simulink model "buckwithmppt"  (R2020b)
settings: Solver=ode23t  StartTime=0.0  StopTime=0.5  RelTol=1e-3
libraries: powerlib x9, re_lib x1, eePwmGenerator x1
settings Model: Creator=shashank Pathak  LastModifiedBy=shashank Pathak

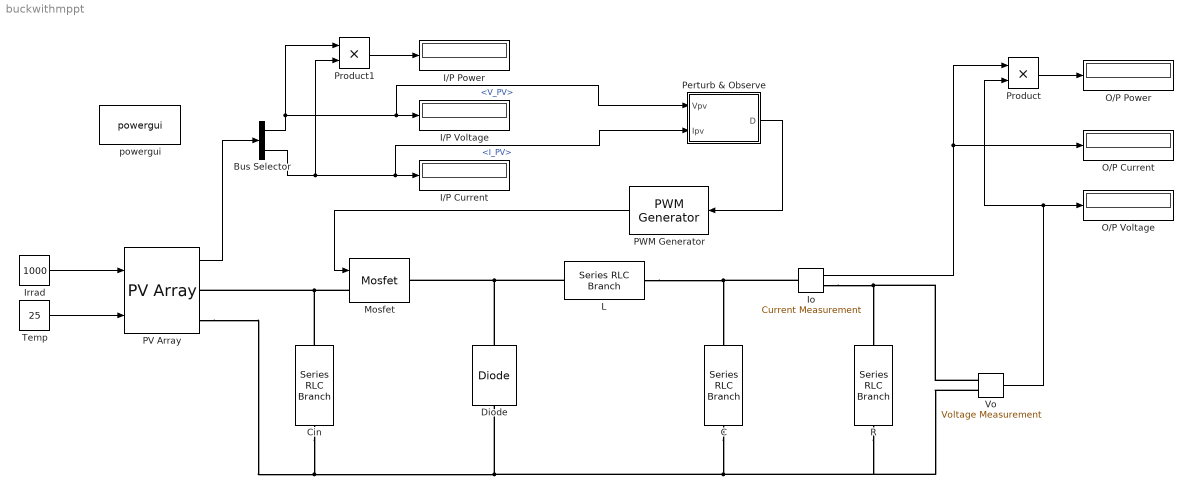
== system buckwithmppt ==
  Bus Selector : BusSelector  OutputSignals=V_PV,I_PV
  C : powerlib/Elements/Series RLC Branch  LConnTagsString=__new0  RConnTagsString=__new0  BranchType=C  Resistance=1  Inductance=1e-3  SetiL0=off  InitialCurrent=0  Capacitance=2.502e-6  Setx0=off  InitialVoltage=0  Measurements=None
  Cin : powerlib/Elements/Series RLC Branch  LConnTagsString=__new0  RConnTagsString=__new0  BranchType=RC  Resistance=0.0001  Inductance=1e-3  SetiL0=off  InitialCurrent=0  Capacitance=1000e-6  Setx0=off  InitialVoltage=0  Measurements=None
  Diode : powerlib/Power Electronics/Diode  Ron=0.001  Lon=0  Vf=0.8  IC=0  UseSnubber=0  Rs=500  Cs=250e-9  Measurements=off
  I/P Current : Display
  I/P Power : Display
  I/P Voltage : Display
  Io : powerlib/Measurements/Current Measurement  PhasorSimulation=off  OutputType=Complex  PSBequivalent=0
  Irrad : Constant  Value=1000
  L : powerlib/Elements/Series RLC Branch  LConnTagsString=__new0  RConnTagsString=__new0  BranchType=L  Resistance=1  Inductance=9.92e-5  SetiL0=off  InitialCurrent=0  Capacitance=1e-6  Setx0=off  InitialVoltage=0  Measurements=None
  Mosfet : powerlib/Power Electronics/Mosfet  Ron=0.1  Lon=0  Rd=0.01  Vfd=0  IC=0  Rs=1e5  Cs=inf  Measurements=off
  O/P Current : Display
  O/P Power : Display
  O/P Voltage : Display
  PV Array : re_lib/Solar/PV Array  Npar=1  Nser=1  PlotType=array @ 25 deg.C & specified irradiances  S_vec=[ 1000 500 100 ]  Temp_C_vec="[ 45 25  ]"  ModuleName=User-defined  PlotWhenSelected=off  Pm=213.15  Ncell=60  Voc=36.3  Isc=7.84  Vm=29  Im=7.35  beta_Voc_pc=-0.36099  alpha_Isc_pc=0.102  beta_Voc=-0.13104  alpha_Isc=0.0079968  IL=7.8654  I0=2.9273e-10  nI=0.98119  Rsh=313.0553  Rs=0.39381  RobustModel=off  RobustCellTemperature=313.3991  BAL=on  Tc=1e-6  Tfilter=5e-5
  PWM Generator : eePwmGenerator/PWM Generator  CarrCount=Up  Tper=1/5000  Ts=10e-6
  Perturb & Observe : MATLAB Function  TreatAsAtomicUnit=on
  Product : Product
  Product1 : Product
  R : powerlib/Elements/Series RLC Branch  LConnTagsString=__new0  RConnTagsString=__new0  BranchType=R  Resistance=1  Inductance=1e-3  SetiL0=off  InitialCurrent=0  Capacitance=1e-6  Setx0=off  InitialVoltage=0  Measurements=None
  Temp : Constant  Value=25
  Vo : powerlib/Measurements/Voltage Measurement  PhasorSimulation=off  OutputType=Complex  PSBequivalent=0
  powergui : powerlib/powergui  Priority=1  SimulationMode=Discrete  SampleTime=1e-6  frequency=60  Iterations=50  frequencyindice=0  Pbase=100e6  ErrMax=1e-4  UnitsV=kV  UnitsW=MW  buscounter=0  FunctionMessages=off  echomessages=off  EnableUseOfTLC=off  CurrentSourceSwitches=off  DisableSnubberDevices=off  DisableRonSwitches=off  DisableVfSwitches=off  DisplayEquations=off  AutomaticDiscreteSolvers=off  SolverType=Tustin/Backward Euler (TBE)  Interpol=off  ExternalGateDelay=off  methode=off  Ts=100  x0status=blocks  SPID=on  SwTol=0  HookPort=off  NonlinearTolerance=1e-4  nMaxIteration=100  ContinueOnMaxIteration=off  RestoreLinks=warning  ResistiveCurrentMeasurement=off  Frange=[0:2:500]  Ylog=off  Xlog=on  ShowGrid=off  save=off  variable=ZData  structure=0  ZoomFFT=off  StartTime=0.0  cycles=1  DisplayStyle=1  fundamental=60  FreqAxis=off  MaxFrequency=1000  frequencyindicesteady=1  RmsSteady=1  display=off
  wires:
  Irrad/1 -> PV Array/1
  Temp/1 -> PV Array/2
  PV Array/1 -> Bus Selector/1
  Bus Selector/1 -> Product1/1, I/P Voltage/1, Perturb & Observe/1(Vpv)  "<V_PV>"
  Bus Selector/2 -> Product1/2, Perturb & Observe/2(Ipv), I/P Current/1  "<I_PV>"
  Io/1 -> Product/1, O/P Current/1
  Vo/1 -> Product/2, O/P Voltage/1
  Product/1 -> O/P Power/1
  Product1/1 -> I/P Power/1
  PWM Generator/1 -> Mosfet/1
  Perturb & Observe/1(D) -> PWM Generator/1
  connections:
  Mosfet/LConn1 -- Cin/LConn1 -- PV Array/RConn1
  L/LConn1 -- Mosfet/RConn1 -- Diode/RConn1
  L/RConn1 -- Io/LConn1 -- C/LConn1
  PV Array/RConn2 -- Cin/RConn1 -- R/RConn1 -- Vo/LConn2 -- C/RConn1 -- Diode/LConn1
  Io/RConn1 -- Vo/LConn1 -- R/LConn1

== matlab function buckwithmppt/Perturb & Observe ==
  data: Vpv input; D output; Ipv input
function D = PO(Vpv, Ipv)

persistent Dprev Vprev Pprev

if isempty(Dprev)
    Dprev = 0.5;
    Vprev = 0;
    Pprev = 0;
end
    
delD = 1e-6;
Ppv = Vpv * Ipv;
dP = Ppv - Pprev;
dV = Vpv - Vprev;

if dP ~= 0
    if dP > 0
        if dV > 0
            D = Dprev - delD;
        else
            D = Dprev + delD;
        end
    else
        if dV > 0
            D = Dprev + delD;
        else
            D = Dprev - delD;
        end
    end
else
    D = Dprev;
end

Dprev = D;
Pprev = Ppv;
Vprev = Vpv;

end
